simulink model "accTests"  (R2019a)
settings: Solver=VariableStepAuto  StartTime=0.0  StopTime=25  RelTol=1e-3
libraries: simulink x21, autolibshared x5
(part 2 of 2)

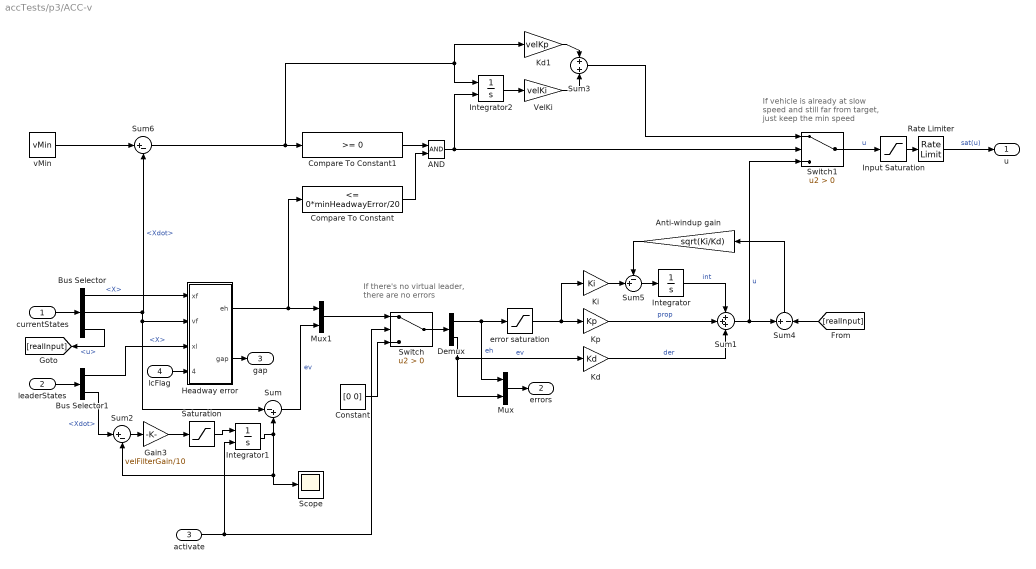
== system accTests/p3/ACC-v ==
  note: If vehicle is already at slow
      | speed and still far from target,
      | just keep the min speed
  note: If there's no virtual leader,
      | there are no errors
  currentStates : Inport
  leaderStates : Inport  Port=2
  activate : Inport  Port=3
  lcFlag : Inport  Port=4
  AND : Logic  IconShape=distinctive  AllPortsSameDT=off  OutDataTypeStr=boolean
  Anti-windup gain : Gain  Gain=sqrt(Ki/Kd)
  Bus Selector : BusSelector  OutputSignals=X,Xdot,u
  Bus Selector1 : BusSelector  OutputSignals=X,Xdot
  Compare To Constant : simulink/Logic and Bit Operations/Compare To Constant  relop=<=  const=0*minHeadwayError/20  OutDataTypeStr=boolean
  Compare To Constant1 : simulink/Logic and Bit Operations/Compare To Constant  relop=>=  const=0  OutDataTypeStr=boolean
  Constant : Constant  Value=[0 0]
  Demux : Demux  Outputs=2
  Gain3 : Gain  Gain=velFilterGain/10
  Headway error : Subsystem
  Input Saturation : Saturate  UpperLimit=maxAcceleration/2  LowerLimit=minAcceleration/4
  Integrator : Integrator
  Integrator1 : Integrator  ExternalReset=rising  InitialCondition=vx0
  Integrator2 : Integrator  ExternalReset=rising
  Kd : Gain  Gain=Kd
  Kd1 : Gain  Gain=velKp
  Ki : Gain  Gain=Ki
  Kp : Gain  Gain=Kp
  Mux : Mux  Inputs=2
  Mux1 : Mux  Inputs=2
  Rate Limiter : RateLimiter  RisingSlewLimit=maxJerk/2  FallingSlewLimit=minJerk/3  SampleTimeMode=inherited
  Saturation : Saturate  UpperLimit=maxAcceleration  LowerLimit=minAcceleration
  Scope : Scope
  Sum : Sum  Inputs=|-+
  Sum1 : Sum  Inputs=+++
  Sum2 : Sum  Inputs=|+-
  Sum3 : Sum
  Sum4 : Sum  Inputs=+-
  Sum5 : Sum  Inputs=-+|
  Sum6 : Sum  Inputs=|+-
  Switch : Switch  Criteria=u2 > Threshold
  Switch1 : Switch  Criteria=u2 > Threshold
  VelKi : Gain  Gain=velKi
  error saturation : Saturate  UpperLimit=maxHeadwayError  LowerLimit=minHeadwayError/10
  vMin : Constant  Value=vMin
  u : Outport
  errors : Outport  Port=2
  gap : Outport  Port=3
  wires:
  Headway error/1(eh) -> Compare To Constant/1, Mux1/1
  Kd/1 -> Sum1/3  "der"
  Kp/1 -> Sum1/2  "prop"
  Gain3/1 -> Saturation/1
  Saturation/1 -> Integrator1/1
  Integrator1/1 -> Scope/1, Sum2/2, Sum/2
  Bus Selector1/2 -> Sum2/1  "<Xdot>"
  Sum2/1 -> Gain3/1
  Demux/1 -> Mux/1, error saturation/1  "eh"
  Headway error/2("gap ") -> gap/1
  Sum1/1 -> Switch1/3, Sum4/1  "u"
  Sum/1 -> Mux1/2  "ev"
  Mux/1 -> errors/1
  Input Saturation/1 -> Rate Limiter/1
  Integrator/1 -> Sum1/1  "int"
  Sum4/1 -> Anti-windup gain/1
  Ki/1 -> Sum5/2
  Anti-windup gain/1 -> Sum5/1
  Demux/2 -> Kd/1, Mux/2  "ev"
  Switch/1 -> Demux/1
  Mux1/1 -> Switch/1
  activate/1 -> Integrator1/2, Switch/2
  Constant/1 -> Switch/3
  Rate Limiter/1 -> u/1  "sat(u)"
  Compare To Constant1/1 -> AND/1
  Compare To Constant/1 -> AND/2
  Sum6/1 -> Integrator2/1, Kd1/1, Compare To Constant1/1
  Sum3/1 -> Switch1/1
  Integrator2/1 -> VelKi/1
  Kd1/1 -> Sum3/1
  VelKi/1 -> Sum3/2
  vMin/1 -> Sum6/1
  Switch1/1 -> Input Saturation/1  "u"
  error saturation/1 -> Kp/1, Ki/1
  Sum5/1 -> Integrator/1
  AND/1 -> Switch1/2, Integrator2/2
  [realInput] -> Sum4/2
  currentStates/1 -> Bus Selector/1
  Bus Selector/1 -> Headway error/1(xf)  "<X>"
  Bus Selector/2 -> Sum6/2, Headway error/2(vf), Sum/1  "<Xdot>"
  leaderStates/1 -> Bus Selector1/1
  Bus Selector1/1 -> Headway error/3(xl)  "<X>"
  Bus Selector/3 -> [realInput]  "<u>"
  lcFlag/1 -> Headway error/4(lcFlag)

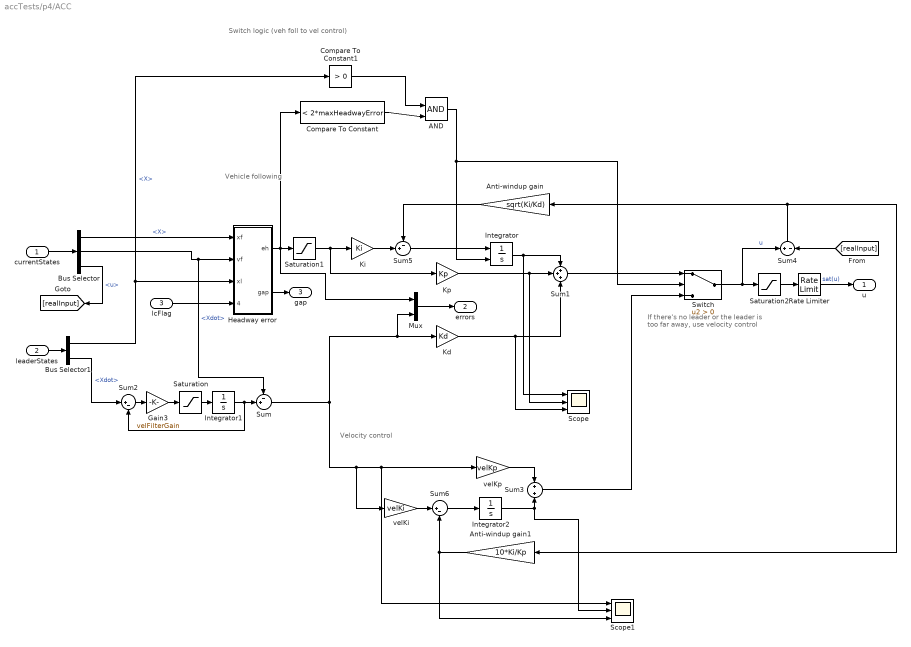
== system accTests/p4/ACC ==
  note: Vehicle following
  note: Switch logic (veh foll to vel control)
  note: Velocity control
  note: If there's no leader or the leader
      | is too far away, use velocity control
  currentStates : Inport
  leaderStates : Inport  Port=2
  lcFlag : Inport  Port=3
  AND : Logic  IconShape=distinctive  AllPortsSameDT=off  OutDataTypeStr=boolean
  Anti-windup gain : Gain  Gain=sqrt(Ki/Kd)
  Anti-windup gain1 : Gain  Gain=10*Ki/Kp
  Bus Selector : BusSelector  OutputSignals=X,Xdot,u
  Bus Selector1 : BusSelector  OutputSignals=X,Xdot
  Compare To Constant : simulink/Logic and Bit Operations/Compare To Constant  relop=<  const=2*maxHeadwayError  OutDataTypeStr=boolean
  Compare To Constant1 : simulink/Logic and Bit Operations/Compare To Constant  relop=>  const=0  OutDataTypeStr=boolean
  Gain3 : Gain  Gain=velFilterGain
  Headway error : Subsystem
  Integrator : Integrator  ExternalReset=either
  Integrator1 : Integrator  InitialCondition=vx0
  Integrator2 : Integrator
  Kd : Gain  Gain=Kd
  Ki : Gain  Gain=Ki
  Kp : Gain  Gain=Kp
  Mux : Mux  Inputs=2
  Rate Limiter : RateLimiter  RisingSlewLimit=maxJerk  FallingSlewLimit=minJerk  SampleTimeMode=inherited
  Saturation : Saturate  UpperLimit=maxAcceleration  LowerLimit=minAcceleration
  Saturation1 : Saturate  UpperLimit=maxHeadwayError  LowerLimit=minHeadwayError
  Saturation2 : Saturate  UpperLimit=maxAcceleration  LowerLimit=minAcceleration
  Scope : Scope  NumInputPorts=3
  Scope1 : Scope  NumInputPorts=3
  Sum : Sum  Inputs=-+|
  Sum1 : Sum  Inputs=+++
  Sum2 : Sum  Inputs=|+-
  Sum3 : Sum
  Sum4 : Sum  Inputs=+-
  Sum5 : Sum  Inputs=-+|
  Sum6 : Sum  Inputs=|+-
  Switch : Switch  Criteria=u2 > Threshold
  velKi : Gain  Gain=velKi
  velKp : Gain  Gain=velKp
  u : Outport
  errors : Outport  Port=2
  gap : Outport  Port=3
  wires:
  Headway error/1(eh) -> Mux/1, Compare To Constant/1, Saturation1/1
  Bus Selector/2 -> Headway error/2(vf), Sum/1  "<Xdot>"
  Kd/1 -> Scope/3, Sum1/3
  Kp/1 -> Scope/2, Sum1/2
  Gain3/1 -> Saturation/1
  Saturation/1 -> Integrator1/1
  Integrator1/1 -> Sum2/2, Sum/2
  Bus Selector1/2 -> Sum2/1  "<Xdot>"
  Sum2/1 -> Gain3/1
  Saturation1/1 -> Kp/1, Ki/1
  Headway error/2("gap ") -> gap/1
  Switch/1 -> Sum4/1, Saturation2/1  "u"
  Sum1/1 -> Switch/1
  Sum3/1 -> Switch/3
  Sum/1 -> Mux/2, Kd/1, velKi/1, Scope1/1, velKp/1
  Mux/1 -> errors/1
  Saturation2/1 -> Rate Limiter/1
  Sum4/1 -> Anti-windup gain/1, Anti-windup gain1/1
  Sum5/1 -> Integrator/1
  Rate Limiter/1 -> u/1  "sat(u)"
  velKp/1 -> Sum3/1
  Ki/1 -> Sum5/2
  Integrator/1 -> Sum1/1, Scope/1
  Anti-windup gain/1 -> Sum5/1
  AND/1 -> Integrator/2, Switch/2
  Compare To Constant/1 -> AND/2
  Compare To Constant1/1 -> AND/1
  lcFlag/1 -> Headway error/4(lcFlag)
  currentStates/1 -> Bus Selector/1
  Bus Selector/1 -> Headway error/1(xf)  "<X>"
  leaderStates/1 -> Bus Selector1/1
  Bus Selector1/1 -> Compare To Constant1/1, Headway error/3(xl)  "<X>"
  Bus Selector/3 -> [realInput]  "<u>"
  [realInput] -> Sum4/2
  Integrator2/1 -> Scope1/2, Sum3/2
  velKi/1 -> Sum6/1
  Sum6/1 -> Integrator2/1
  Anti-windup gain1/1 -> Scope1/3, Sum6/2

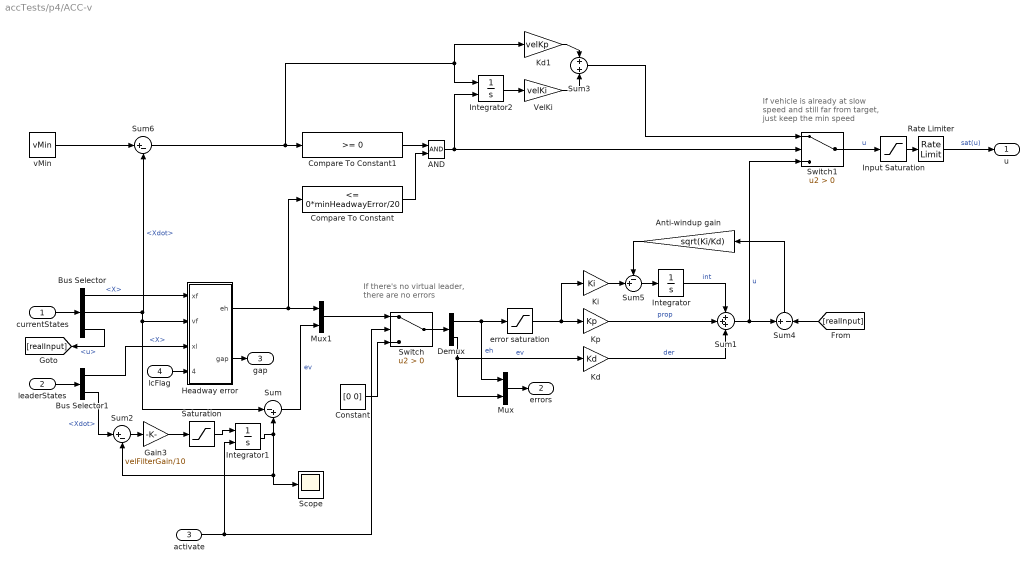
== system accTests/p4/ACC-v ==
  note: If vehicle is already at slow
      | speed and still far from target,
      | just keep the min speed
  note: If there's no virtual leader,
      | there are no errors
  currentStates : Inport
  leaderStates : Inport  Port=2
  activate : Inport  Port=3
  lcFlag : Inport  Port=4
  AND : Logic  IconShape=distinctive  AllPortsSameDT=off  OutDataTypeStr=boolean
  Anti-windup gain : Gain  Gain=sqrt(Ki/Kd)
  Bus Selector : BusSelector  OutputSignals=X,Xdot,u
  Bus Selector1 : BusSelector  OutputSignals=X,Xdot
  Compare To Constant : simulink/Logic and Bit Operations/Compare To Constant  relop=<=  const=0*minHeadwayError/20  OutDataTypeStr=boolean
  Compare To Constant1 : simulink/Logic and Bit Operations/Compare To Constant  relop=>=  const=0  OutDataTypeStr=boolean
  Constant : Constant  Value=[0 0]
  Demux : Demux  Outputs=2
  Gain3 : Gain  Gain=velFilterGain/10
  Headway error : Subsystem
  Input Saturation : Saturate  UpperLimit=maxAcceleration/2  LowerLimit=minAcceleration/4
  Integrator : Integrator
  Integrator1 : Integrator  ExternalReset=rising  InitialCondition=vx0
  Integrator2 : Integrator  ExternalReset=rising
  Kd : Gain  Gain=Kd
  Kd1 : Gain  Gain=velKp
  Ki : Gain  Gain=Ki
  Kp : Gain  Gain=Kp
  Mux : Mux  Inputs=2
  Mux1 : Mux  Inputs=2
  Rate Limiter : RateLimiter  RisingSlewLimit=maxJerk/2  FallingSlewLimit=minJerk/3  SampleTimeMode=inherited
  Saturation : Saturate  UpperLimit=maxAcceleration  LowerLimit=minAcceleration
  Scope : Scope
  Sum : Sum  Inputs=|-+
  Sum1 : Sum  Inputs=+++
  Sum2 : Sum  Inputs=|+-
  Sum3 : Sum
  Sum4 : Sum  Inputs=+-
  Sum5 : Sum  Inputs=-+|
  Sum6 : Sum  Inputs=|+-
  Switch : Switch  Criteria=u2 > Threshold
  Switch1 : Switch  Criteria=u2 > Threshold
  VelKi : Gain  Gain=velKi
  error saturation : Saturate  UpperLimit=maxHeadwayError  LowerLimit=minHeadwayError/10
  vMin : Constant  Value=vMin
  u : Outport
  errors : Outport  Port=2
  gap : Outport  Port=3
  wires:
  Headway error/1(eh) -> Compare To Constant/1, Mux1/1
  Kd/1 -> Sum1/3  "der"
  Kp/1 -> Sum1/2  "prop"
  Gain3/1 -> Saturation/1
  Saturation/1 -> Integrator1/1
  Integrator1/1 -> Scope/1, Sum2/2, Sum/2
  Bus Selector1/2 -> Sum2/1  "<Xdot>"
  Sum2/1 -> Gain3/1
  Demux/1 -> Mux/1, error saturation/1  "eh"
  Headway error/2("gap ") -> gap/1
  Sum1/1 -> Switch1/3, Sum4/1  "u"
  Sum/1 -> Mux1/2  "ev"
  Mux/1 -> errors/1
  Input Saturation/1 -> Rate Limiter/1
  Integrator/1 -> Sum1/1  "int"
  Sum4/1 -> Anti-windup gain/1
  Ki/1 -> Sum5/2
  Anti-windup gain/1 -> Sum5/1
  Demux/2 -> Kd/1, Mux/2  "ev"
  Switch/1 -> Demux/1
  Mux1/1 -> Switch/1
  activate/1 -> Integrator1/2, Switch/2
  Constant/1 -> Switch/3
  Rate Limiter/1 -> u/1  "sat(u)"
  Compare To Constant1/1 -> AND/1
  Compare To Constant/1 -> AND/2
  Sum6/1 -> Integrator2/1, Kd1/1, Compare To Constant1/1
  Sum3/1 -> Switch1/1
  Integrator2/1 -> VelKi/1
  Kd1/1 -> Sum3/1
  VelKi/1 -> Sum3/2
  vMin/1 -> Sum6/1
  Switch1/1 -> Input Saturation/1  "u"
  error saturation/1 -> Kp/1, Ki/1
  Sum5/1 -> Integrator/1
  AND/1 -> Switch1/2, Integrator2/2
  [realInput] -> Sum4/2
  currentStates/1 -> Bus Selector/1
  Bus Selector/1 -> Headway error/1(xf)  "<X>"
  Bus Selector/2 -> Sum6/2, Headway error/2(vf), Sum/1  "<Xdot>"
  leaderStates/1 -> Bus Selector1/1
  Bus Selector1/1 -> Headway error/3(xl)  "<X>"
  Bus Selector/3 -> [realInput]  "<u>"
  lcFlag/1 -> Headway error/4(lcFlag)

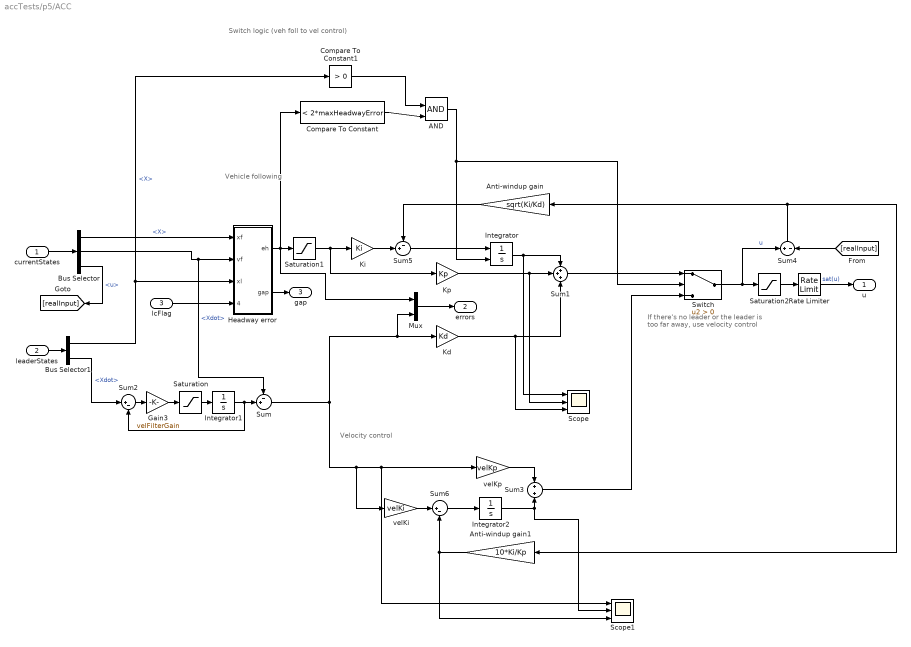
== system accTests/p5/ACC ==
  note: Vehicle following
  note: Switch logic (veh foll to vel control)
  note: Velocity control
  note: If there's no leader or the leader
      | is too far away, use velocity control
  currentStates : Inport
  leaderStates : Inport  Port=2
  lcFlag : Inport  Port=3
  AND : Logic  IconShape=distinctive  AllPortsSameDT=off  OutDataTypeStr=boolean
  Anti-windup gain : Gain  Gain=sqrt(Ki/Kd)
  Anti-windup gain1 : Gain  Gain=10*Ki/Kp
  Bus Selector : BusSelector  OutputSignals=X,Xdot,u
  Bus Selector1 : BusSelector  OutputSignals=X,Xdot
  Compare To Constant : simulink/Logic and Bit Operations/Compare To Constant  relop=<  const=2*maxHeadwayError  OutDataTypeStr=boolean
  Compare To Constant1 : simulink/Logic and Bit Operations/Compare To Constant  relop=>  const=0  OutDataTypeStr=boolean
  Gain3 : Gain  Gain=velFilterGain
  Headway error : Subsystem
  Integrator : Integrator  ExternalReset=either
  Integrator1 : Integrator  InitialCondition=vx0
  Integrator2 : Integrator
  Kd : Gain  Gain=Kd
  Ki : Gain  Gain=Ki
  Kp : Gain  Gain=Kp
  Mux : Mux  Inputs=2
  Rate Limiter : RateLimiter  RisingSlewLimit=maxJerk  FallingSlewLimit=minJerk  SampleTimeMode=inherited
  Saturation : Saturate  UpperLimit=maxAcceleration  LowerLimit=minAcceleration
  Saturation1 : Saturate  UpperLimit=maxHeadwayError  LowerLimit=minHeadwayError
  Saturation2 : Saturate  UpperLimit=maxAcceleration  LowerLimit=minAcceleration
  Scope : Scope  NumInputPorts=3
  Scope1 : Scope  NumInputPorts=3
  Sum : Sum  Inputs=-+|
  Sum1 : Sum  Inputs=+++
  Sum2 : Sum  Inputs=|+-
  Sum3 : Sum
  Sum4 : Sum  Inputs=+-
  Sum5 : Sum  Inputs=-+|
  Sum6 : Sum  Inputs=|+-
  Switch : Switch  Criteria=u2 > Threshold
  velKi : Gain  Gain=velKi
  velKp : Gain  Gain=velKp
  u : Outport
  errors : Outport  Port=2
  gap : Outport  Port=3
  wires:
  Headway error/1(eh) -> Mux/1, Compare To Constant/1, Saturation1/1
  Bus Selector/2 -> Headway error/2(vf), Sum/1  "<Xdot>"
  Kd/1 -> Scope/3, Sum1/3
  Kp/1 -> Scope/2, Sum1/2
  Gain3/1 -> Saturation/1
  Saturation/1 -> Integrator1/1
  Integrator1/1 -> Sum2/2, Sum/2
  Bus Selector1/2 -> Sum2/1  "<Xdot>"
  Sum2/1 -> Gain3/1
  Saturation1/1 -> Kp/1, Ki/1
  Headway error/2("gap ") -> gap/1
  Switch/1 -> Sum4/1, Saturation2/1  "u"
  Sum1/1 -> Switch/1
  Sum3/1 -> Switch/3
  Sum/1 -> Mux/2, Kd/1, velKi/1, Scope1/1, velKp/1
  Mux/1 -> errors/1
  Saturation2/1 -> Rate Limiter/1
  Sum4/1 -> Anti-windup gain/1, Anti-windup gain1/1
  Sum5/1 -> Integrator/1
  Rate Limiter/1 -> u/1  "sat(u)"
  velKp/1 -> Sum3/1
  Ki/1 -> Sum5/2
  Integrator/1 -> Sum1/1, Scope/1
  Anti-windup gain/1 -> Sum5/1
  AND/1 -> Integrator/2, Switch/2
  Compare To Constant/1 -> AND/2
  Compare To Constant1/1 -> AND/1
  lcFlag/1 -> Headway error/4(lcFlag)
  currentStates/1 -> Bus Selector/1
  Bus Selector/1 -> Headway error/1(xf)  "<X>"
  leaderStates/1 -> Bus Selector1/1
  Bus Selector1/1 -> Compare To Constant1/1, Headway error/3(xl)  "<X>"
  Bus Selector/3 -> [realInput]  "<u>"
  [realInput] -> Sum4/2
  Integrator2/1 -> Scope1/2, Sum3/2
  velKi/1 -> Sum6/1
  Sum6/1 -> Integrator2/1
  Anti-windup gain1/1 -> Scope1/3, Sum6/2

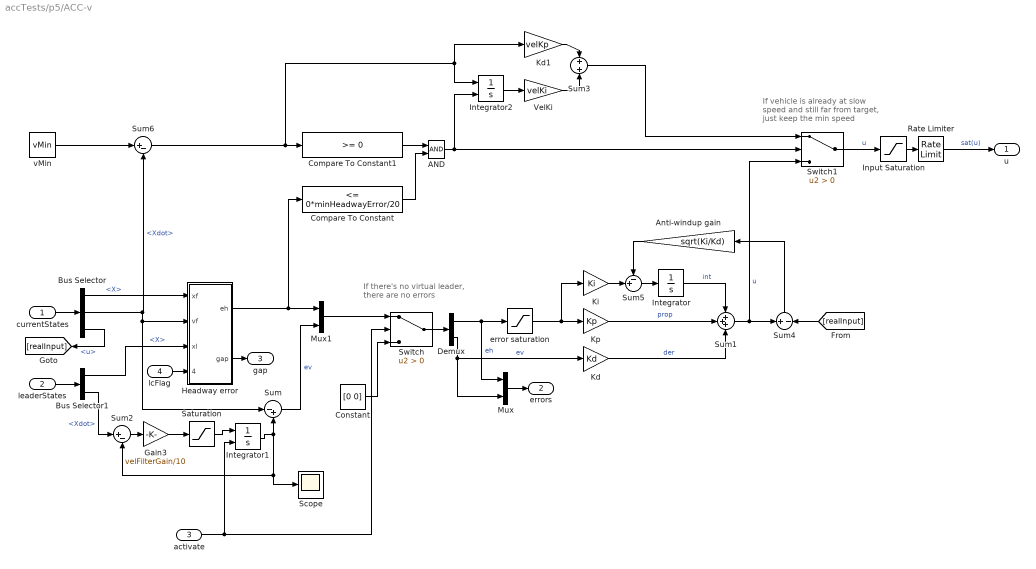
== system accTests/p5/ACC-v ==
  note: If vehicle is already at slow
      | speed and still far from target,
      | just keep the min speed
  note: If there's no virtual leader,
      | there are no errors
  currentStates : Inport
  leaderStates : Inport  Port=2
  activate : Inport  Port=3
  lcFlag : Inport  Port=4
  AND : Logic  IconShape=distinctive  AllPortsSameDT=off  OutDataTypeStr=boolean
  Anti-windup gain : Gain  Gain=sqrt(Ki/Kd)
  Bus Selector : BusSelector  OutputSignals=X,Xdot,u
  Bus Selector1 : BusSelector  OutputSignals=X,Xdot
  Compare To Constant : simulink/Logic and Bit Operations/Compare To Constant  relop=<=  const=0*minHeadwayError/20  OutDataTypeStr=boolean
  Compare To Constant1 : simulink/Logic and Bit Operations/Compare To Constant  relop=>=  const=0  OutDataTypeStr=boolean
  Constant : Constant  Value=[0 0]
  Demux : Demux  Outputs=2
  Gain3 : Gain  Gain=velFilterGain/10
  Headway error : Subsystem
  Input Saturation : Saturate  UpperLimit=maxAcceleration/2  LowerLimit=minAcceleration/4
  Integrator : Integrator
  Integrator1 : Integrator  ExternalReset=rising  InitialCondition=vx0
  Integrator2 : Integrator  ExternalReset=rising
  Kd : Gain  Gain=Kd
  Kd1 : Gain  Gain=velKp
  Ki : Gain  Gain=Ki
  Kp : Gain  Gain=Kp
  Mux : Mux  Inputs=2
  Mux1 : Mux  Inputs=2
  Rate Limiter : RateLimiter  RisingSlewLimit=maxJerk/2  FallingSlewLimit=minJerk/3  SampleTimeMode=inherited
  Saturation : Saturate  UpperLimit=maxAcceleration  LowerLimit=minAcceleration
  Scope : Scope
  Sum : Sum  Inputs=|-+
  Sum1 : Sum  Inputs=+++
  Sum2 : Sum  Inputs=|+-
  Sum3 : Sum
  Sum4 : Sum  Inputs=+-
  Sum5 : Sum  Inputs=-+|
  Sum6 : Sum  Inputs=|+-
  Switch : Switch  Criteria=u2 > Threshold
  Switch1 : Switch  Criteria=u2 > Threshold
  VelKi : Gain  Gain=velKi
  error saturation : Saturate  UpperLimit=maxHeadwayError  LowerLimit=minHeadwayError/10
  vMin : Constant  Value=vMin
  u : Outport
  errors : Outport  Port=2
  gap : Outport  Port=3
  wires:
  Headway error/1(eh) -> Compare To Constant/1, Mux1/1
  Kd/1 -> Sum1/3  "der"
  Kp/1 -> Sum1/2  "prop"
  Gain3/1 -> Saturation/1
  Saturation/1 -> Integrator1/1
  Integrator1/1 -> Scope/1, Sum2/2, Sum/2
  Bus Selector1/2 -> Sum2/1  "<Xdot>"
  Sum2/1 -> Gain3/1
  Demux/1 -> Mux/1, error saturation/1  "eh"
  Headway error/2("gap ") -> gap/1
  Sum1/1 -> Switch1/3, Sum4/1  "u"
  Sum/1 -> Mux1/2  "ev"
  Mux/1 -> errors/1
  Input Saturation/1 -> Rate Limiter/1
  Integrator/1 -> Sum1/1  "int"
  Sum4/1 -> Anti-windup gain/1
  Ki/1 -> Sum5/2
  Anti-windup gain/1 -> Sum5/1
  Demux/2 -> Kd/1, Mux/2  "ev"
  Switch/1 -> Demux/1
  Mux1/1 -> Switch/1
  activate/1 -> Integrator1/2, Switch/2
  Constant/1 -> Switch/3
  Rate Limiter/1 -> u/1  "sat(u)"
  Compare To Constant1/1 -> AND/1
  Compare To Constant/1 -> AND/2
  Sum6/1 -> Integrator2/1, Kd1/1, Compare To Constant1/1
  Sum3/1 -> Switch1/1
  Integrator2/1 -> VelKi/1
  Kd1/1 -> Sum3/1
  VelKi/1 -> Sum3/2
  vMin/1 -> Sum6/1
  Switch1/1 -> Input Saturation/1  "u"
  error saturation/1 -> Kp/1, Ki/1
  Sum5/1 -> Integrator/1
  AND/1 -> Switch1/2, Integrator2/2
  [realInput] -> Sum4/2
  currentStates/1 -> Bus Selector/1
  Bus Selector/1 -> Headway error/1(xf)  "<X>"
  Bus Selector/2 -> Sum6/2, Headway error/2(vf), Sum/1  "<Xdot>"
  leaderStates/1 -> Bus Selector1/1
  Bus Selector1/1 -> Headway error/3(xl)  "<X>"
  Bus Selector/3 -> [realInput]  "<u>"
  lcFlag/1 -> Headway error/4(lcFlag)

== system accTests/p1/ACC/Headway error ==
  xf : Inport
  vf : Inport  Port=2
  xl : Inport  Port=3
  lcFlag : Inport  Port=4
  Demux : Demux  Outputs=2
  Gain : Gain  Gain=0.5
  Integrator : Integrator  InitialCondition=[h d0]
  Multiply : Product
  Mux : Mux  Inputs=2
  Mux1 : Mux  Inputs=2
  Sum : Sum  Inputs=-+|
  Sum1 : Sum  Inputs=++|
  Sum2 : Sum  Inputs=+-|
  Sum3 : Sum  Inputs=|++
  Sum4 : Sum  Inputs=|+-
  Switch : Switch  Criteria=u2 > Threshold
  d0 : Constant  Value=d0
  d0Lc : Constant  Value=d0Lc
  h : Constant  Value=h
  hLc : Constant  Value=hLc
  vLen : Constant  Value=lr+lf
  eh : Outport
  "gap " : Outport  Port=2
  wires:
  vLen/1 -> Sum1/1
  Multiply/1 -> Sum3/1
  Sum/1 -> "gap "/1, Sum2/1  "gap"
  xf/1 -> Sum1/2
  Sum3/1 -> Sum2/2  "desired  gap"
  vf/1 -> Multiply/1
  Sum1/1 -> Sum/1  "x (front bumber)"
  xl/1 -> Sum/2
  h/1 -> Mux/1
  Switch/1 -> Sum4/1
  Gain/1 -> Integrator/1
  Sum4/1 -> Gain/1
  Integrator/1 -> Sum4/2, Demux/1
  lcFlag/1 -> Switch/2
  Sum2/1 -> eh/1
  d0/1 -> Mux/2
  Mux/1 -> Switch/3
  hLc/1 -> Mux1/1
  d0Lc/1 -> Mux1/2
  Mux1/1 -> Switch/1
  Demux/1 -> Multiply/2  "time headway"
  Demux/2 -> Sum3/2  "gap at  standstill"

== system accTests/p1/ACC-v/Headway error ==
  xf : Inport
  vf : Inport  Port=2
  xl : Inport  Port=3
  lcFlag : Inport  Port=4
  Demux : Demux  Outputs=2
  Gain : Gain  Gain=0.5
  Integrator : Integrator  InitialCondition=h
  Multiply : Product
  Mux : Mux  Inputs=2
  Mux1 : Mux  Inputs=2
  Sum : Sum  Inputs=-+|
  Sum1 : Sum  Inputs=++|
  Sum2 : Sum  Inputs=+-|
  Sum3 : Sum  Inputs=|++
  Sum4 : Sum  Inputs=|+-
  Switch : Switch  Criteria=u2 > Threshold
  d0 : Constant  Value=d0
  d0Lc : Constant  Value=d0Lc
  h : Constant  Value=h
  hLc : Constant  Value=hLc
  vLen : Constant  Value=lr+lf
  eh : Outport
  "gap " : Outport  Port=2
  wires:
  vLen/1 -> Sum1/1
  Multiply/1 -> Sum3/1
  Sum/1 -> "gap "/1, Sum2/1  "gap"
  xf/1 -> Sum1/2
  Sum3/1 -> Sum2/2  "desired  gap"
  vf/1 -> Multiply/1
  Sum1/1 -> Sum/1  "x (front bumber)"
  xl/1 -> Sum/2
  h/1 -> Mux/1
  Switch/1 -> Sum4/1
  Gain/1 -> Integrator/1
  Sum4/1 -> Gain/1
  Integrator/1 -> Sum4/2, Demux/1
  lcFlag/1 -> Switch/2
  Sum2/1 -> eh/1
  d0/1 -> Mux/2
  Mux/1 -> Switch/3
  hLc/1 -> Mux1/1
  d0Lc/1 -> Mux1/2
  Mux1/1 -> Switch/1
  Demux/1 -> Multiply/2  "time headway"
  Demux/2 -> Sum3/2  "gap at  standstill"

== system accTests/p2/ACC/Headway error ==
  xf : Inport
  vf : Inport  Port=2
  xl : Inport  Port=3
  lcFlag : Inport  Port=4
  Demux : Demux  Outputs=2
  Gain : Gain  Gain=0.5
  Integrator : Integrator  InitialCondition=[h d0]
  Multiply : Product
  Mux : Mux  Inputs=2
  Mux1 : Mux  Inputs=2
  Sum : Sum  Inputs=-+|
  Sum1 : Sum  Inputs=++|
  Sum2 : Sum  Inputs=+-|
  Sum3 : Sum  Inputs=|++
  Sum4 : Sum  Inputs=|+-
  Switch : Switch  Criteria=u2 > Threshold
  d0 : Constant  Value=d0
  d0Lc : Constant  Value=d0Lc
  h : Constant  Value=h
  hLc : Constant  Value=hLc
  vLen : Constant  Value=lr+lf
  eh : Outport
  "gap " : Outport  Port=2
  wires:
  vLen/1 -> Sum1/1
  Multiply/1 -> Sum3/1
  Sum/1 -> "gap "/1, Sum2/1  "gap"
  xf/1 -> Sum1/2
  Sum3/1 -> Sum2/2  "desired  gap"
  vf/1 -> Multiply/1
  Sum1/1 -> Sum/1  "x (front bumber)"
  xl/1 -> Sum/2
  h/1 -> Mux/1
  Switch/1 -> Sum4/1
  Gain/1 -> Integrator/1
  Sum4/1 -> Gain/1
  Integrator/1 -> Sum4/2, Demux/1
  lcFlag/1 -> Switch/2
  Sum2/1 -> eh/1
  d0/1 -> Mux/2
  Mux/1 -> Switch/3
  hLc/1 -> Mux1/1
  d0Lc/1 -> Mux1/2
  Mux1/1 -> Switch/1
  Demux/1 -> Multiply/2  "time headway"
  Demux/2 -> Sum3/2  "gap at  standstill"

== system accTests/p2/ACC-v/Headway error ==
  xf : Inport
  vf : Inport  Port=2
  xl : Inport  Port=3
  lcFlag : Inport  Port=4
  Demux : Demux  Outputs=2
  Gain : Gain  Gain=0.5
  Integrator : Integrator  InitialCondition=h
  Multiply : Product
  Mux : Mux  Inputs=2
  Mux1 : Mux  Inputs=2
  Sum : Sum  Inputs=-+|
  Sum1 : Sum  Inputs=++|
  Sum2 : Sum  Inputs=+-|
  Sum3 : Sum  Inputs=|++
  Sum4 : Sum  Inputs=|+-
  Switch : Switch  Criteria=u2 > Threshold
  d0 : Constant  Value=d0
  d0Lc : Constant  Value=d0Lc
  h : Constant  Value=h
  hLc : Constant  Value=hLc
  vLen : Constant  Value=lr+lf
  eh : Outport
  "gap " : Outport  Port=2
  wires:
  vLen/1 -> Sum1/1
  Multiply/1 -> Sum3/1
  Sum/1 -> "gap "/1, Sum2/1  "gap"
  xf/1 -> Sum1/2
  Sum3/1 -> Sum2/2  "desired  gap"
  vf/1 -> Multiply/1
  Sum1/1 -> Sum/1  "x (front bumber)"
  xl/1 -> Sum/2
  h/1 -> Mux/1
  Switch/1 -> Sum4/1
  Gain/1 -> Integrator/1
  Sum4/1 -> Gain/1
  Integrator/1 -> Sum4/2, Demux/1
  lcFlag/1 -> Switch/2
  Sum2/1 -> eh/1
  d0/1 -> Mux/2
  Mux/1 -> Switch/3
  hLc/1 -> Mux1/1
  d0Lc/1 -> Mux1/2
  Mux1/1 -> Switch/1
  Demux/1 -> Multiply/2  "time headway"
  Demux/2 -> Sum3/2  "gap at  standstill"

== system accTests/p3/ACC/Headway error ==
  xf : Inport
  vf : Inport  Port=2
  xl : Inport  Port=3
  lcFlag : Inport  Port=4
  Demux : Demux  Outputs=2
  Gain : Gain  Gain=0.5
  Integrator : Integrator  InitialCondition=[h d0]
  Multiply : Product
  Mux : Mux  Inputs=2
  Mux1 : Mux  Inputs=2
  Sum : Sum  Inputs=-+|
  Sum1 : Sum  Inputs=++|
  Sum2 : Sum  Inputs=+-|
  Sum3 : Sum  Inputs=|++
  Sum4 : Sum  Inputs=|+-
  Switch : Switch  Criteria=u2 > Threshold
  d0 : Constant  Value=d0
  d0Lc : Constant  Value=d0Lc
  h : Constant  Value=h
  hLc : Constant  Value=hLc
  vLen : Constant  Value=lr+lf
  eh : Outport
  "gap " : Outport  Port=2
  wires:
  vLen/1 -> Sum1/1
  Multiply/1 -> Sum3/1
  Sum/1 -> "gap "/1, Sum2/1  "gap"
  xf/1 -> Sum1/2
  Sum3/1 -> Sum2/2  "desired  gap"
  vf/1 -> Multiply/1
  Sum1/1 -> Sum/1  "x (front bumber)"
  xl/1 -> Sum/2
  h/1 -> Mux/1
  Switch/1 -> Sum4/1
  Gain/1 -> Integrator/1
  Sum4/1 -> Gain/1
  Integrator/1 -> Sum4/2, Demux/1
  lcFlag/1 -> Switch/2
  Sum2/1 -> eh/1
  d0/1 -> Mux/2
  Mux/1 -> Switch/3
  hLc/1 -> Mux1/1
  d0Lc/1 -> Mux1/2
  Mux1/1 -> Switch/1
  Demux/1 -> Multiply/2  "time headway"
  Demux/2 -> Sum3/2  "gap at  standstill"

== system accTests/p3/ACC-v/Headway error ==
  xf : Inport
  vf : Inport  Port=2
  xl : Inport  Port=3
  lcFlag : Inport  Port=4
  Demux : Demux  Outputs=2
  Gain : Gain  Gain=0.5
  Integrator : Integrator  InitialCondition=h
  Multiply : Product
  Mux : Mux  Inputs=2
  Mux1 : Mux  Inputs=2
  Sum : Sum  Inputs=-+|
  Sum1 : Sum  Inputs=++|
  Sum2 : Sum  Inputs=+-|
  Sum3 : Sum  Inputs=|++
  Sum4 : Sum  Inputs=|+-
  Switch : Switch  Criteria=u2 > Threshold
  d0 : Constant  Value=d0
  d0Lc : Constant  Value=d0Lc
  h : Constant  Value=h
  hLc : Constant  Value=hLc
  vLen : Constant  Value=lr+lf
  eh : Outport
  "gap " : Outport  Port=2
  wires:
  vLen/1 -> Sum1/1
  Multiply/1 -> Sum3/1
  Sum/1 -> "gap "/1, Sum2/1  "gap"
  xf/1 -> Sum1/2
  Sum3/1 -> Sum2/2  "desired  gap"
  vf/1 -> Multiply/1
  Sum1/1 -> Sum/1  "x (front bumber)"
  xl/1 -> Sum/2
  h/1 -> Mux/1
  Switch/1 -> Sum4/1
  Gain/1 -> Integrator/1
  Sum4/1 -> Gain/1
  Integrator/1 -> Sum4/2, Demux/1
  lcFlag/1 -> Switch/2
  Sum2/1 -> eh/1
  d0/1 -> Mux/2
  Mux/1 -> Switch/3
  hLc/1 -> Mux1/1
  d0Lc/1 -> Mux1/2
  Mux1/1 -> Switch/1
  Demux/1 -> Multiply/2  "time headway"
  Demux/2 -> Sum3/2  "gap at  standstill"

== system accTests/p4/ACC/Headway error ==
  xf : Inport
  vf : Inport  Port=2
  xl : Inport  Port=3
  lcFlag : Inport  Port=4
  Demux : Demux  Outputs=2
  Gain : Gain  Gain=0.5
  Integrator : Integrator  InitialCondition=[h d0]
  Multiply : Product
  Mux : Mux  Inputs=2
  Mux1 : Mux  Inputs=2
  Sum : Sum  Inputs=-+|
  Sum1 : Sum  Inputs=++|
  Sum2 : Sum  Inputs=+-|
  Sum3 : Sum  Inputs=|++
  Sum4 : Sum  Inputs=|+-
  Switch : Switch  Criteria=u2 > Threshold
  d0 : Constant  Value=d0
  d0Lc : Constant  Value=d0Lc
  h : Constant  Value=h
  hLc : Constant  Value=hLc
  vLen : Constant  Value=lr+lf
  eh : Outport
  "gap " : Outport  Port=2
  wires:
  vLen/1 -> Sum1/1
  Multiply/1 -> Sum3/1
  Sum/1 -> "gap "/1, Sum2/1  "gap"
  xf/1 -> Sum1/2
  Sum3/1 -> Sum2/2  "desired  gap"
  vf/1 -> Multiply/1
  Sum1/1 -> Sum/1  "x (front bumber)"
  xl/1 -> Sum/2
  h/1 -> Mux/1
  Switch/1 -> Sum4/1
  Gain/1 -> Integrator/1
  Sum4/1 -> Gain/1
  Integrator/1 -> Sum4/2, Demux/1
  lcFlag/1 -> Switch/2
  Sum2/1 -> eh/1
  d0/1 -> Mux/2
  Mux/1 -> Switch/3
  hLc/1 -> Mux1/1
  d0Lc/1 -> Mux1/2
  Mux1/1 -> Switch/1
  Demux/1 -> Multiply/2  "time headway"
  Demux/2 -> Sum3/2  "gap at  standstill"

== system accTests/p4/ACC-v/Headway error ==
  xf : Inport
  vf : Inport  Port=2
  xl : Inport  Port=3
  lcFlag : Inport  Port=4
  Demux : Demux  Outputs=2
  Gain : Gain  Gain=0.5
  Integrator : Integrator  InitialCondition=h
  Multiply : Product
  Mux : Mux  Inputs=2
  Mux1 : Mux  Inputs=2
  Sum : Sum  Inputs=-+|
  Sum1 : Sum  Inputs=++|
  Sum2 : Sum  Inputs=+-|
  Sum3 : Sum  Inputs=|++
  Sum4 : Sum  Inputs=|+-
  Switch : Switch  Criteria=u2 > Threshold
  d0 : Constant  Value=d0
  d0Lc : Constant  Value=d0Lc
  h : Constant  Value=h
  hLc : Constant  Value=hLc
  vLen : Constant  Value=lr+lf
  eh : Outport
  "gap " : Outport  Port=2
  wires:
  vLen/1 -> Sum1/1
  Multiply/1 -> Sum3/1
  Sum/1 -> "gap "/1, Sum2/1  "gap"
  xf/1 -> Sum1/2
  Sum3/1 -> Sum2/2  "desired  gap"
  vf/1 -> Multiply/1
  Sum1/1 -> Sum/1  "x (front bumber)"
  xl/1 -> Sum/2
  h/1 -> Mux/1
  Switch/1 -> Sum4/1
  Gain/1 -> Integrator/1
  Sum4/1 -> Gain/1
  Integrator/1 -> Sum4/2, Demux/1
  lcFlag/1 -> Switch/2
  Sum2/1 -> eh/1
  d0/1 -> Mux/2
  Mux/1 -> Switch/3
  hLc/1 -> Mux1/1
  d0Lc/1 -> Mux1/2
  Mux1/1 -> Switch/1
  Demux/1 -> Multiply/2  "time headway"
  Demux/2 -> Sum3/2  "gap at  standstill"

== system accTests/p5/ACC/Headway error ==
  xf : Inport
  vf : Inport  Port=2
  xl : Inport  Port=3
  lcFlag : Inport  Port=4
  Demux : Demux  Outputs=2
  Gain : Gain  Gain=0.5
  Integrator : Integrator  InitialCondition=[h d0]
  Multiply : Product
  Mux : Mux  Inputs=2
  Mux1 : Mux  Inputs=2
  Sum : Sum  Inputs=-+|
  Sum1 : Sum  Inputs=++|
  Sum2 : Sum  Inputs=+-|
  Sum3 : Sum  Inputs=|++
  Sum4 : Sum  Inputs=|+-
  Switch : Switch  Criteria=u2 > Threshold
  d0 : Constant  Value=d0
  d0Lc : Constant  Value=d0Lc
  h : Constant  Value=h
  hLc : Constant  Value=hLc
  vLen : Constant  Value=lr+lf
  eh : Outport
  "gap " : Outport  Port=2
  wires:
  vLen/1 -> Sum1/1
  Multiply/1 -> Sum3/1
  Sum/1 -> "gap "/1, Sum2/1  "gap"
  xf/1 -> Sum1/2
  Sum3/1 -> Sum2/2  "desired  gap"
  vf/1 -> Multiply/1
  Sum1/1 -> Sum/1  "x (front bumber)"
  xl/1 -> Sum/2
  h/1 -> Mux/1
  Switch/1 -> Sum4/1
  Gain/1 -> Integrator/1
  Sum4/1 -> Gain/1
  Integrator/1 -> Sum4/2, Demux/1
  lcFlag/1 -> Switch/2
  Sum2/1 -> eh/1
  d0/1 -> Mux/2
  Mux/1 -> Switch/3
  hLc/1 -> Mux1/1
  d0Lc/1 -> Mux1/2
  Mux1/1 -> Switch/1
  Demux/1 -> Multiply/2  "time headway"
  Demux/2 -> Sum3/2  "gap at  standstill"

== system accTests/p5/ACC-v/Headway error ==
  xf : Inport
  vf : Inport  Port=2
  xl : Inport  Port=3
  lcFlag : Inport  Port=4
  Demux : Demux  Outputs=2
  Gain : Gain  Gain=0.5
  Integrator : Integrator  InitialCondition=h
  Multiply : Product
  Mux : Mux  Inputs=2
  Mux1 : Mux  Inputs=2
  Sum : Sum  Inputs=-+|
  Sum1 : Sum  Inputs=++|
  Sum2 : Sum  Inputs=+-|
  Sum3 : Sum  Inputs=|++
  Sum4 : Sum  Inputs=|+-
  Switch : Switch  Criteria=u2 > Threshold
  d0 : Constant  Value=d0
  d0Lc : Constant  Value=d0Lc
  h : Constant  Value=h
  hLc : Constant  Value=hLc
  vLen : Constant  Value=lr+lf
  eh : Outport
  "gap " : Outport  Port=2
  wires:
  vLen/1 -> Sum1/1
  Multiply/1 -> Sum3/1
  Sum/1 -> "gap "/1, Sum2/1  "gap"
  xf/1 -> Sum1/2
  Sum3/1 -> Sum2/2  "desired  gap"
  vf/1 -> Multiply/1
  Sum1/1 -> Sum/1  "x (front bumber)"
  xl/1 -> Sum/2
  h/1 -> Mux/1
  Switch/1 -> Sum4/1
  Gain/1 -> Integrator/1
  Sum4/1 -> Gain/1
  Integrator/1 -> Sum4/2, Demux/1
  lcFlag/1 -> Switch/2
  Sum2/1 -> eh/1
  d0/1 -> Mux/2
  Mux/1 -> Switch/3
  hLc/1 -> Mux1/1
  d0Lc/1 -> Mux1/2
  Mux1/1 -> Switch/1
  Demux/1 -> Multiply/2  "time headway"
  Demux/2 -> Sum3/2  "gap at  standstill"
